simulink model "PID_Fuzzy_DauDun_2016a"  (R2016a)
settings: Solver=ode5  SolverMode=SingleTasking  StartTime=0.0  StopTime=400  FixedStep=0.1  MaxStep=0.1  RelTol=1e-3
libraries: fuzblock x1
Description:
  | The model describes dynamic properties of tank level system. The differential equation is:
  |                                            d/dt{Ah(t))=ku(t)-a*sqrt(2*g*h(t))
settings Model: ExtModeTrigMode=oneshot  ExtModeArmWhenConnect=off  Creator=Huynh Thai Hoang  LastModifiedBy=ASUS
settings SolverCC: InitialStep=0.1
settings DataIOCC: SaveFormat=Array  SignalLoggingSaveFormat=ModelDataLogs  SaveOutput=off  SaveTime=off  SignalLoggingName=sigsOut
settings OptimizationCC: BooleanDataType=off  ExpressionDepthLimit=2147483647
settings DebuggingCC: SaveWithParameterizedLinksMsg=none  UnderspecifiedInitializationDetection=Classic  MergeDetectMultiDrivingBlocksExec=none  SignalResolutionControl=TryResolveAllWithWarning  MultiTaskDSMMsg=warning  MultiTaskCondExecSysMsg=none  FcnCallInpInsideContextMsg=EnableAllAsWarning  StateNameClashWarn=warning
settings HardwareCC: ProdBitPerPointer=32  ProdLargestAtomicFloat=None  ProdIntDivRoundTo=Undefined  ProdEndianess=Unspecified  ProdWordSize=32  ProdHWDeviceType=32-bit Generic  TargetBitPerPointer=64  TargetLongLongMode=on  TargetIntDivRoundTo=Zero  TargetEndianess=LittleEndian  TargetWordSize=64  TargetHWDeviceType=MATLAB Host  ProdEqTarget=off
settings ModelReferenceCC: PropagateSignalLabelsOutOfModel=off
settings GRTTargetCC: CombineOutputUpdateFcns=off  GRTInterface=on

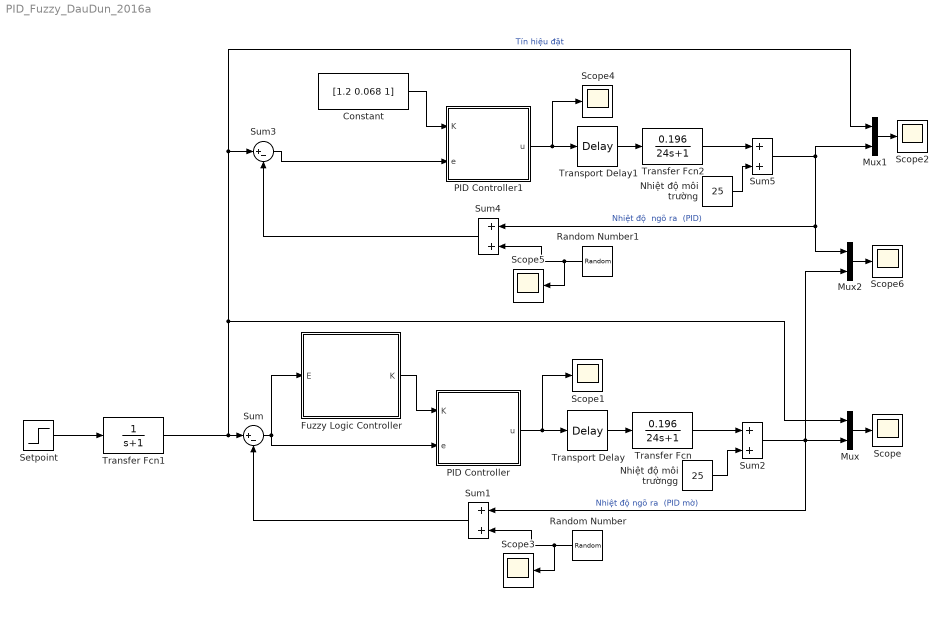
== system PID_Fuzzy_DauDun_2016a ==
  Constant : Constant  Value=[1.2 0.068 1]
  Fuzzy Logic Controller : Subsystem
  Mux : Mux  Inputs=2
  Mux1 : Mux  Inputs=2
  Mux2 : Mux  Inputs=2
  Nhiệt độ môi trường : Constant  Value=25
  Nhiệt độ môi trườngg : Constant  Value=25
  PID Controller : Subsystem  AncestorBlock=simulink_extras/Additional Linear/PID Controller  mask(PID Controller){}
      mask help:
      | Enter expressions for proportional, integral, and derivative terms.
      | P+I/s+Ds
      mask Help: This block implements a PID controller where parameters are entered for the Proportional, Integral and Derivative terms. Unmask this block to see how it works. The derivative term is implemented using a true derivative block.
  PID Controller1 : Subsystem  AncestorBlock=simulink_extras/Additional Linear/PID Controller  mask(PID Controller){}
      mask help:
      | Enter expressions for proportional, integral, and derivative terms.
      | P+I/s+Ds
      mask Help: This block implements a PID controller where parameters are entered for the Proportional, Integral and Derivative terms. Unmask this block to see how it works. The derivative term is implemented using a true derivative block.
  Random Number : RandomNumber  Variance=0.1
  Random Number1 : RandomNumber  Variance=0.1
  Scope{,1..6} (7 alike) : Scope
  Setpoint : Step  Time=20.7  Before=25  After=360  SampleTime=0
  Sum : Sum  Inputs=|+-  SaturateOnIntegerOverflow=on
  Sum{1..2,4..5} (4 alike) : Sum  SaturateOnIntegerOverflow=on
  Sum3 : Sum  Inputs=|+-  SaturateOnIntegerOverflow=on
  Transfer Fcn : TransferFcn  Numerator=[0.196]  Denominator=[24 1]
  Transfer Fcn1 : TransferFcn  Denominator=[1 1]
  Transfer Fcn2 : TransferFcn  Numerator=[0.196]  Denominator=[24 1]
  Transport Delay : TransportDelay  DelayTime=20.7
  Transport Delay1 : TransportDelay  DelayTime=20.7
  wires:
  Sum/1 -> Fuzzy Logic Controller/1(E), PID Controller/2(e)
  PID Controller/1(u) -> Transport Delay/1, Scope1/1
  Mux/1 -> Scope/1
  Transport Delay/1 -> Transfer Fcn/1
  Sum1/1 -> Sum/2
  Transfer Fcn/1 -> Sum2/1
  Sum2/1 -> Mux2/2, Mux/2, Sum1/1  "Nhiệt độ ngõ ra  (PID mờ)"
  Nhiệt độ môi trườngg/1 -> Sum2/2
  Random Number/1 -> Scope3/1, Sum1/2
  Fuzzy Logic Controller/1(K) -> PID Controller/1(K)
  Constant/1 -> PID Controller1/1(K)
  Transfer Fcn1/1 -> Mux/1, Sum3/1, Mux1/1, Sum/1  "Tín hiệu đặt"
  Random Number1/1 -> Sum4/2, Scope5/1
  Nhiệt độ môi trường/1 -> Sum5/2
  Sum5/1 -> Mux1/2, Mux2/1, Sum4/1  "Nhiệt độ  ngõ ra  (PID)"
  Transfer Fcn2/1 -> Sum5/1
  Sum4/1 -> Sum3/2
  Transport Delay1/1 -> Transfer Fcn2/1
  Mux1/1 -> Scope2/1
  PID Controller1/1(u) -> Scope4/1, Transport Delay1/1
  Sum3/1 -> PID Controller1/2(e)
  Mux2/1 -> Scope6/1
  Setpoint/1 -> Transfer Fcn1/1

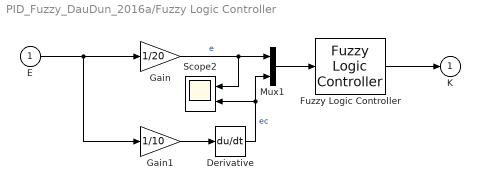
== system PID_Fuzzy_DauDun_2016a/Fuzzy Logic Controller ==
  E : Inport
  Derivative : Derivative
  Fuzzy Logic Controller : fuzblock/Fuzzy Logic  Controller  FIS='PID_Control.fis'
  Gain : Gain  Gain=1/20
  Gain1 : Gain  Gain=1/10
  Mux1 : Mux  Inputs=2
  Scope2 : Scope  NumInputPorts=2
  K : Outport
  wires:
  Fuzzy Logic Controller/1 -> K/1
  Gain/1 -> Mux1/1, Scope2/1  "e"
  Derivative/1 -> Mux1/2, Scope2/2  "ec"
  Gain1/1 -> Derivative/1
  E/1 -> Gain1/1, Gain/1
  Mux1/1 -> Fuzzy Logic Controller/1

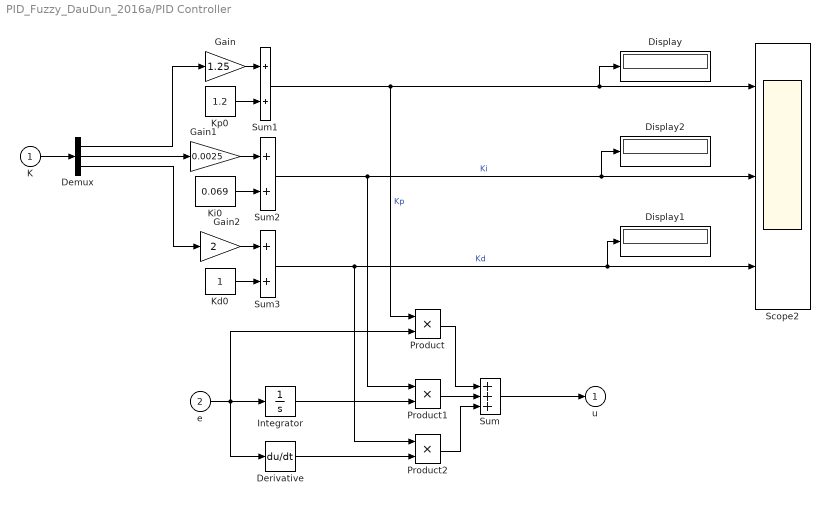
== system PID_Fuzzy_DauDun_2016a/PID Controller ==
  K : Inport
  e : Inport  Port=2
  Demux : Demux  Outputs=3
  Derivative : Derivative
  Display : Display
  Display1 : Display
  Display2 : Display
  Gain : Gain  Gain=1.25
  Gain1 : Gain  Gain=0.0025
  Gain2 : Gain  Gain=2
  Integrator : Integrator
  Kd0 : Constant
  Ki0 : Constant  Value=0.069
  Kp0 : Constant  Value=1.2
  Product : Product  SaturateOnIntegerOverflow=on  OutDataTypeStr=Inherit: Same as first input
  Product1 : Product  SaturateOnIntegerOverflow=on  OutDataTypeStr=Inherit: Same as first input
  Product2 : Product  SaturateOnIntegerOverflow=on  OutDataTypeStr=Inherit: Same as first input
  Scope2 : Scope  NumInputPorts=3
  Sum : Sum  Inputs=+++  SaturateOnIntegerOverflow=on  InputSameDT=on  OutDataTypeStr=Inherit: Same as first input
  Sum1 : Sum  SaturateOnIntegerOverflow=on  InputSameDT=on  OutDataTypeStr=Inherit: Same as first input
  Sum2 : Sum  SaturateOnIntegerOverflow=on  InputSameDT=on  OutDataTypeStr=Inherit: Same as first input
  Sum3 : Sum  SaturateOnIntegerOverflow=on  InputSameDT=on  OutDataTypeStr=Inherit: Same as first input
  u : Outport  InitialOutput=0
  wires:
  Product/1 -> Sum/1
  e/1 -> Product/2, Integrator/1, Derivative/1
  K/1 -> Demux/1
  Product1/1 -> Sum/2
  Integrator/1 -> Product1/2
  Derivative/1 -> Product2/2
  Product2/1 -> Sum/3
  Sum/1 -> u/1
  Kp0/1 -> Sum1/2
  Kd0/1 -> Sum3/2
  Ki0/1 -> Sum2/2
  Gain1/1 -> Sum2/1
  Gain2/1 -> Sum3/1
  Demux/1 -> Gain/1
  Gain/1 -> Sum1/1
  Demux/2 -> Gain1/1
  Demux/3 -> Gain2/1
  Sum2/1 -> Product1/1, Display2/1, Scope2/2  "Ki"
  Sum3/1 -> Display1/1, Scope2/3, Product2/1  "Kd"
  Sum1/1 -> Display/1, Scope2/1, Product/1  "Kp"

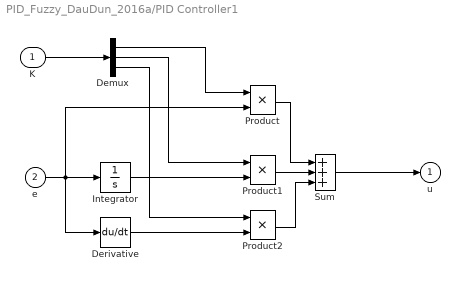
== system PID_Fuzzy_DauDun_2016a/PID Controller1 ==
  K : Inport
  e : Inport  Port=2
  Demux : Demux  Outputs=3
  Derivative : Derivative
  Integrator : Integrator
  Product : Product  SaturateOnIntegerOverflow=on  OutDataTypeStr=Inherit: Same as first input
  Product1 : Product  SaturateOnIntegerOverflow=on  OutDataTypeStr=Inherit: Same as first input
  Product2 : Product  SaturateOnIntegerOverflow=on  OutDataTypeStr=Inherit: Same as first input
  Sum : Sum  Inputs=+++  SaturateOnIntegerOverflow=on  InputSameDT=on  OutDataTypeStr=Inherit: Same as first input
  u : Outport  InitialOutput=0
  wires:
  Demux/3 -> Product2/1
  Demux/2 -> Product1/1
  Demux/1 -> Product/1
  Sum/1 -> u/1
  Product2/1 -> Sum/3
  Derivative/1 -> Product2/2
  Integrator/1 -> Product1/2
  Product1/1 -> Sum/2
  K/1 -> Demux/1
  e/1 -> Derivative/1, Integrator/1, Product/2
  Product/1 -> Sum/1
